simulink model "be3"  (R2013a)
settings: Solver=ode45  StartTime=0.0  StopTime=10.0  RelTol=1e-3
values from neighbouring files (symbols this model uses):
  A = -f0/J    (= -4.5652173913)    [variablesCC.m]
  B = Km/J    (= 652.173913043)    [variablesCC.m]
  C = 1    [variablesCC.m]
  f1 = 3 * 10^(-4)    (= 0.0003)    [variablesCC.m]
  g13 = Kr3 / (zbp3 - 1)    [variablesCC.m]
  J = 9.2 * 10^(-5)    (= 9.2e-05)    [variablesCC.m]
  Kr3 = K3(2)    [variablesCC.m]
  Kt3 = K3(1)    [variablesCC.m]
  Te = 250*10^(-6)    (= 0.00025)    [variablesCC.m]
settings Model: Creator=tfumey  LastModifiedBy=tfumey

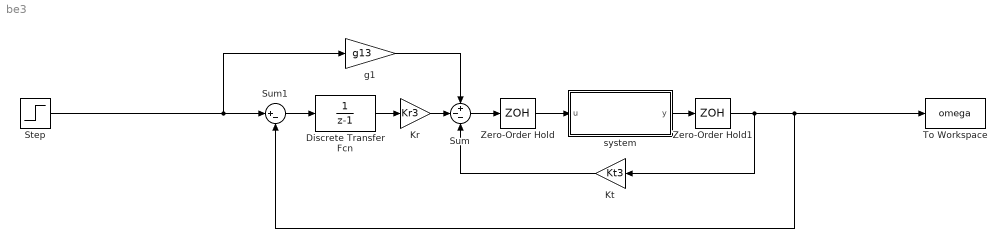
== system be3 ==
  Discrete Transfer Fcn : DiscreteTransferFcn  Denominator=[1 -1]  SampleTime=Te
  Kr : Gain  Gain=Kr3
  "Kt " : Gain  Gain=Kt3
  Step : Step  SampleTime=0
  Sum : Sum  Inputs=+--
  Sum1 : Sum  Inputs=|+-
  To Workspace : ToWorkspace  VariableName=omega  SampleTime=-1  SaveFormat=Timeseries
  Zero-Order Hold : ZeroOrderHold  SampleTime=Te
  Zero-Order Hold1 : ZeroOrderHold  SampleTime=Te
  g1 : Gain  Gain=g13
  system : Subsystem
  wires:
  Kr/1 -> Sum/2
  Discrete Transfer Fcn/1 -> Kr/1
  Sum1/1 -> Discrete Transfer Fcn/1
  g1/1 -> Sum/1
  Step/1 -> Sum1/1, g1/1
  Zero-Order Hold/1 -> system/1(u)
  Sum/1 -> Zero-Order Hold/1
  "Kt "/1 -> Sum/3
  system/1(y) -> Zero-Order Hold1/1
  Zero-Order Hold1/1 -> Sum1/2, To Workspace/1, "Kt "/1

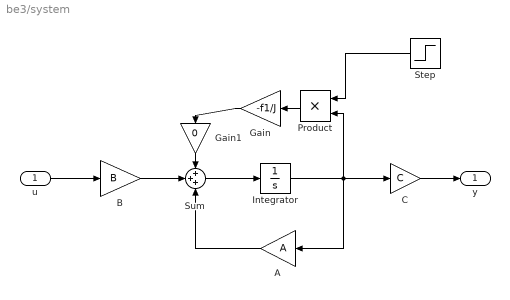
== system be3/system ==
  u : Inport
  A : Gain  Gain=A
  B : Gain  Gain=B
  C : Gain  Gain=C
  Gain : Gain  Gain=-f1/J
  Gain1 : Gain  Gain=0
  Integrator : Integrator
  Product : Product
  Step : Step  Time=1.1  SampleTime=0
  Sum : Sum  Inputs=+++
  y : Outport
  wires:
  u/1 -> B/1
  Sum/1 -> Integrator/1
  Integrator/1 -> Product/2, C/1, A/1
  C/1 -> y/1
  A/1 -> Sum/3
  B/1 -> Sum/2
  Gain/1 -> Gain1/1
  Product/1 -> Gain/1
  Step/1 -> Product/1
  Gain1/1 -> Sum/1
